simulink model "SingleStreamSSR"  (R2019b)
settings: Solver=VariableStepAuto  StartTime=0.0  StopTime=500  RelTol=1e-3
PreLoadFcn:
  | SSR4_init;
InitFcn:
  | xmcCheckSlxPath(bdroot)
  | SSR4_init;
values from neighbouring files (symbols this model uses):
  SHIFT_ACC = 15    [SSR4_init.m]
  Taps = NormalizeCoef(UTaps,32768)    [SSR4_init.m]
undefined symbols (not defined in the file or in its folder): FIR_MultiKernel_cin, FIR_MultiKernel_cincout, FIR_MultiKernel_cout, SingleStream, xc7vx485tffg1157
libraries: ModelComposer x37, dspsrcs4 x1
(part 1 of 2)
settings Model: Creator=oliviert  LastModifiedBy=abehbood

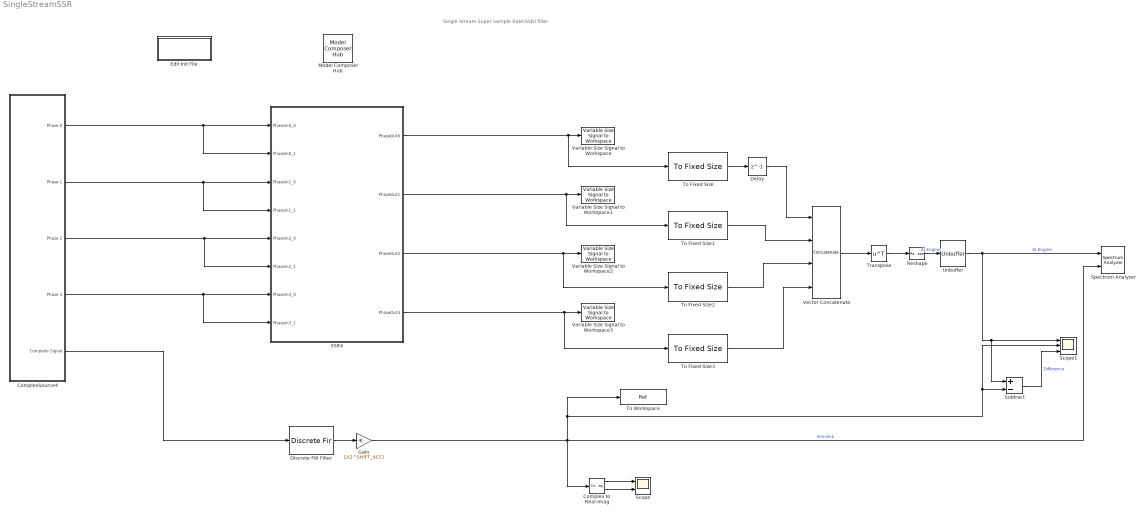
== system SingleStreamSSR ==
  note: Single Stream Super Sample Rate(SSR) filter
  Complex to Real-Imag : ComplexToRealImag
  ComplexSource4 : Subsystem  mask{s=0}
      mask prompts: s "Seed"
  Delay : Delay  DelayLength=1
  Discrete FIR Filter : DiscreteFir  Coefficients=Taps  InputProcessing=Columns as channels (frame based)
  Edit Init File : Subsystem
      settings: OpenFcn=edit('SSR4_init.m');
  Gain : Gain  Gain=1/(2^SHIFT_ACC)
  Model Composer Hub : ModelComposer/Model Composer Hub  CodeGeneration=off  SubsystemName=SSR4  TargetDirectory=./code_kernel  ExportType=AI Engines  IpVendor=xilinx.com  IpLibrary=hls  IpVersion=1.0  IpHWLanguage=Verilog  AieCompilerOptions={}  CreateTestbench=on  TestbenchStackSize=10  RunAieSim=on  AieSimTimeout=5000  LaunchVitisAnalyzer=off  PlotOutput=off  RunX86Sim=off  X86SimTimeout=10  ProjDevice=xc7vx485tffg1157-1  ProjDevicePart=xc7vx485tffg1157-1  SamplePeriod=-1  ClockFrequency=200  DataPathParallelism=1
  Reshape : Reshape
  SSR4 : Subsystem
  Scope : Scope  NumInputPorts=2
  Scope1 : Scope  NumInputPorts=3
  Spectrum Analyzer : SpectrumAnalyzer  NumInputPorts=2
  Subtract : Sum  Inputs=+-
  To Fixed Size{,1..3} (4 alike) : ModelComposer/To Fixed Size  OutputSize=4  HasStatusOutput=off
  To Workspace : ToWorkspace  VariableName=Ref  SampleTime=-1
      settings: Save2DSignal=2-D array (concatenate along first dimension)
  Transpose : Math  Operator=transpose  SignedPower=off  SaturateOnIntegerOverflow=on
  Unbuffer : Unbuffer
  Variable Size Signal to Workspace : ModelComposer/Variable Size Signal to Workspace  VariableNameMask=P0
  Variable Size Signal to Workspace1 : ModelComposer/Variable Size Signal to Workspace  VariableNameMask=P1
  Variable Size Signal to Workspace2 : ModelComposer/Variable Size Signal to Workspace  VariableNameMask=P2
  Variable Size Signal to Workspace3 : ModelComposer/Variable Size Signal to Workspace  VariableNameMask=P3
  Vector Concatenate : Concatenate  NumInputs=4  Mode=Multidimensional array  ConcatenateDimension=2
  wires:
  Discrete FIR Filter/1 -> Gain/1
  ComplexSource4/5(Complete Signal) -> Discrete FIR Filter/1
  Gain/1 -> Spectrum Analyzer/2, Subtract/2, Scope1/2, To Workspace/1, Complex to Real-Imag/1  "Simulink"
  Complex to Real-Imag/2 -> Scope/2
  Complex to Real-Imag/1 -> Scope/1
  ComplexSource4/1(Phase 0) -> SSR4/2(PhaseIn0_1), SSR4/1(PhaseIn0_0)
  ComplexSource4/2(Phase 1) -> SSR4/4(PhaseIn1_1), SSR4/3(PhaseIn1_0)
  ComplexSource4/3(Phase 2) -> SSR4/6(PhaseIn2_1), SSR4/5(PhaseIn2_0)
  ComplexSource4/4(Phase 3) -> SSR4/8(PhaseIn3_1), SSR4/7(PhaseIn3_0)
  To Fixed Size/1 -> Delay/1
  To Fixed Size1/1 -> Vector Concatenate/2
  To Fixed Size2/1 -> Vector Concatenate/3
  To Fixed Size3/1 -> Vector Concatenate/4
  Vector Concatenate/1 -> Transpose/1
  Transpose/1 -> Reshape/1
  Delay/1 -> Vector Concatenate/1
  Reshape/1 -> Unbuffer/1  "AI Engine"
  Unbuffer/1 -> Subtract/1, Scope1/1, Spectrum Analyzer/1  "AI Engine"
  Subtract/1 -> Scope1/3  "Difference"
  SSR4/1(PhaseOut0) -> To Fixed Size/1, Variable Size Signal to Workspace/1
  SSR4/2(PhaseOut1) -> To Fixed Size1/1, Variable Size Signal to Workspace1/1
  SSR4/3(PhaseOut2) -> To Fixed Size2/1, Variable Size Signal to Workspace2/1
  SSR4/4(PhaseOut3) -> To Fixed Size3/1, Variable Size Signal to Workspace3/1

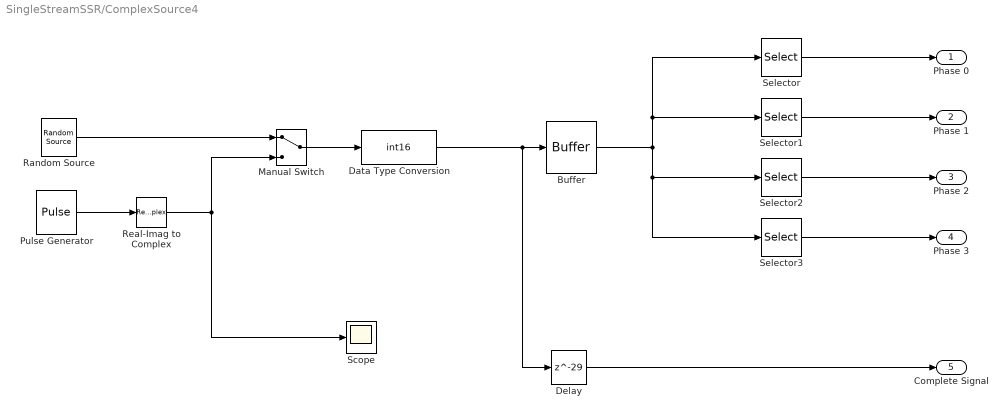
== system SingleStreamSSR/ComplexSource4 ==
  Buffer : Buffer  N=16  OutputFrames=off
  Data Type Conversion : DataTypeConversion  OutDataTypeStr=int16
  Delay : Delay  DelayLength=29
  Manual Switch : ManualSwitch
  Pulse Generator : DiscretePulseGenerator  Period=32 + 40*5  PhaseDelay=32  SampleTime=1/8
  Random Source : dspsrcs4/Random Source  SrcType=Uniform  NormMethod=Ziggurat  CltLength=12  MinVal=-20000  MaxVal=20000  MeanVal=0  VarVal=1  RepMode=Specify seed  rawSeed=s  IsInherit=off  SampMode=Discrete  SampTime=1/8  SampFrame=1  DataType=Double  OutComplex=Complex  OutputFrames=off
  Real-Imag to Complex : RealImagToComplex  Input=Real
  Scope : Scope
  Selector : Selector  InputPortWidth=16  IndexOptions=Index vector (dialog)  Indices=[1:4:16]  OutputSizes=1
  Selector1 : Selector  InputPortWidth=16  IndexOptions=Index vector (dialog)  Indices=[2:4:16]  OutputSizes=1
  Selector2 : Selector  InputPortWidth=16  IndexOptions=Index vector (dialog)  Indices=[3:4:16]  OutputSizes=1
  Selector3 : Selector  InputPortWidth=16  IndexOptions=Index vector (dialog)  Indices=[4:4:16]  OutputSizes=1
  Phase 0 : Outport
  Phase 1 : Outport  Port=2
  Phase 2 : Outport  Port=3
  Phase 3 : Outport  Port=4
  Complete Signal : Outport  Port=5
  wires:
  Selector/1 -> Phase 0/1
  Selector1/1 -> Phase 1/1
  Selector2/1 -> Phase 2/1
  Selector3/1 -> Phase 3/1
  Manual Switch/1 -> Data Type Conversion/1
  Random Source/1 -> Manual Switch/1
  Buffer/1 -> Selector1/1, Selector/1, Selector2/1, Selector3/1
  Real-Imag to Complex/1 -> Scope/1, Manual Switch/2
  Delay/1 -> Complete Signal/1
  Data Type Conversion/1 -> Delay/1, Buffer/1
  Pulse Generator/1 -> Real-Imag to Complex/1

== system SingleStreamSSR/Edit Init File ==
